simulink model "buck4ph_averaged"  (R2024a)
settings: Solver=ode23tb  StartTime=0.0  StopTime=0.001  MaxStep=1.9999999999999999e-07  RelTol=0.0001
undefined symbols (not defined in the file): load_end_a, load_start_a, slew_a_per_us, step_trigger_s, temp_c
settings Model: Creator=ejliixa  LastModifiedBy=ejliixa

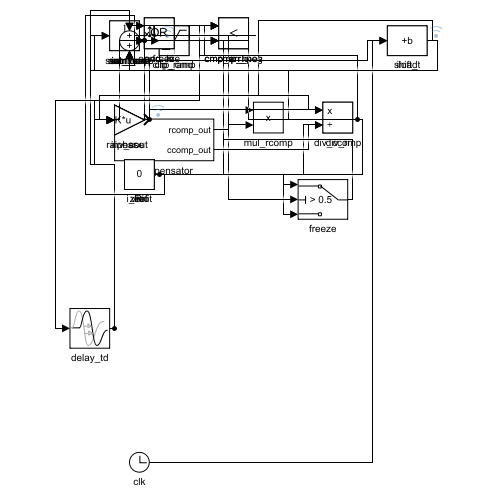
[thumbnail: Simulink's stored preview of the top-level diagram]
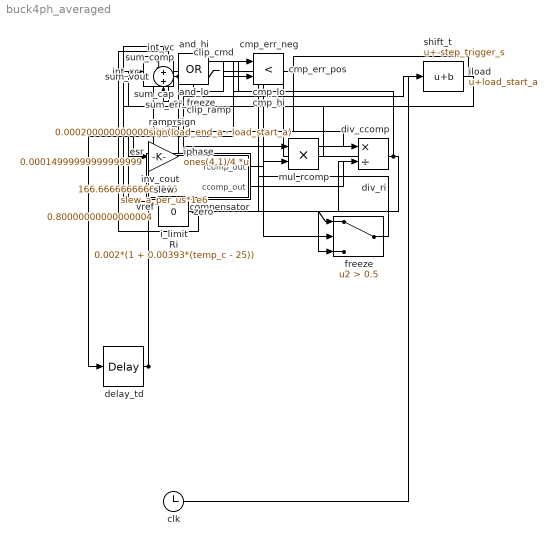
== system buck4ph_averaged ==
  Ri : Constant  Value=0.002*(1 + 0.00393*(temp_c - 25))
  and_hi : Logic  AllPortsSameDT=off  OutDataTypeStr=boolean
  and_lo : Logic  AllPortsSameDT=off  OutDataTypeStr=boolean
  clip_cmd : Saturate  UpperLimit=300  LowerLimit=0
  clip_ramp : Saturate  UpperLimit=abs(load_end_a - load_start_a)  LowerLimit=0
  clk : Clock
  cmp_err_neg : RelationalOperator  Operator=<  OutDataTypeStr=boolean  RndMeth=Simplest  InputSameDT=off
  cmp_err_pos : RelationalOperator  Operator=>  OutDataTypeStr=boolean  RndMeth=Simplest  InputSameDT=off
  cmp_hi : RelationalOperator  Operator=>  OutDataTypeStr=boolean  RndMeth=Simplest  InputSameDT=off
  cmp_lo : RelationalOperator  Operator=<  OutDataTypeStr=boolean  RndMeth=Simplest  InputSameDT=off
  compensator : Subsystem
  delay_td : TransportDelay  DelayTime=2.4999999999999999e-07  InitialOutput=load_start_a
  div_ccomp : Product  Inputs=*/
  div_ri : Product  Inputs=*/
  esr : Gain  Gain=0.00014999999999999999
  freeze : Switch  Criteria=u2 > Threshold  Threshold=0.5  SaturateOnIntegerOverflow=off  InputSameDT=off
  gm : Gain  Gain=0.00020000000000000001
  i_limit : Constant  Value=300
  iload : Bias  Bias=load_start_a  SaturateOnIntegerOverflow=off
  int_vc : Integrator  InitialCondition=0.80000000000000004
  int_xc : Integrator  InitialCondition=load_start_a*(0.002*(1 + 0.00393*(temp_c - 25)))
  inv_cout : Gain  Gain=166.66666666666666
  iphase : Gain  Gain=ones(4,1)/4  Multiplication=Matrix(K*u)
  mul_rcomp : Product
  or_freeze : Logic  Operator=OR  AllPortsSameDT=off  OutDataTypeStr=boolean
  ramp_sign : Gain  Gain=sign(load_end_a - load_start_a)
  shift_t : Bias  Bias=-step_trigger_s  SaturateOnIntegerOverflow=off
  slew : Gain  Gain=slew_a_per_us*1e6
  sum_cap : Sum  Inputs=+-
  sum_comp : Sum
  sum_err : Sum  Inputs=+-
  sum_vout : Sum
  vref : Constant  Value=0.80000000000000004
  zero : Constant  Value=0
  wires:
  clk/1 -> shift_t/1
  shift_t/1 -> slew/1
  slew/1 -> clip_ramp/1
  clip_ramp/1 -> ramp_sign/1
  ramp_sign/1 -> iload/1
  vref/1 -> sum_err/1
  sum_vout/1 -> sum_err/2
  sum_err/1 -> gm/1, cmp_err_pos/1, cmp_err_neg/1
  gm/1 -> mul_rcomp/1, div_ccomp/1
  compensator/1(rcomp_out) -> mul_rcomp/2
  compensator/2(ccomp_out) -> div_ccomp/2
  div_ccomp/1 -> freeze/3
  zero/1 -> freeze/1, cmp_lo/2, cmp_err_pos/2, cmp_err_neg/2
  or_freeze/1 -> freeze/2
  freeze/1 -> int_xc/1
  int_xc/1 -> sum_comp/1
  mul_rcomp/1 -> sum_comp/2
  sum_comp/1 -> div_ri/1
  Ri/1 -> div_ri/2
  div_ri/1 -> clip_cmd/1, cmp_hi/1, cmp_lo/1
  i_limit/1 -> cmp_hi/2
  cmp_hi/1 -> and_hi/1
  cmp_err_pos/1 -> and_hi/2
  cmp_lo/1 -> and_lo/1
  cmp_err_neg/1 -> and_lo/2
  and_hi/1 -> or_freeze/1
  and_lo/1 -> or_freeze/2
  clip_cmd/1 -> delay_td/1
  delay_td/1 -> sum_cap/1, iphase/1
  iload/1 -> sum_cap/2
  sum_cap/1 -> inv_cout/1, esr/1
  inv_cout/1 -> int_vc/1
  esr/1 -> sum_vout/1
  int_vc/1 -> sum_vout/2

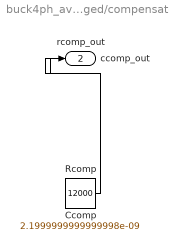
== system buck4ph_averaged/compensator ==
  Ccomp : Constant  Value=2.1999999999999998e-09
  Rcomp : Constant  Value=12000
  rcomp_out : Outport
  ccomp_out : Outport  Port=2
  wires:
  Rcomp/1 -> rcomp_out/1
  Ccomp/1 -> ccomp_out/1
